simulink model "SOC_predict"  (R2023b)
settings: Solver=FixedStepDiscrete  StartTime=0.0  StopTime=timeVector(end)  FixedStep=stepSize  RelTol=1e-3
undefined symbols (not defined in the file): X_MAX, X_MIN
libraries: statsLibrary x1
settings Model: Creator=The MathWorks, Inc.  LastModifiedBy=The MathWorks, Inc.
settings OptimizationCC: BlockReduction=off  ConditionallyExecuteInputs=off  DefaultParameterBehavior=Inlined  InheritOutputTypeSmallerThanSingle=on
settings DebuggingCC: AlgebraicLoopMsg=error  InheritedTsInSrcMsg=none  SingleTaskRateTransMsg=error
settings HardwareCC: ProdBitPerPointer=32  ProdBitPerSizeT=32  ProdBitPerPtrDiffT=32  ProdLargestAtomicFloat=None  ProdIntDivRoundTo=Undefined  ProdEndianess=Unspecified  ProdWordSize=32  ProdHWDeviceType=ASIC/FPGA->ASIC/FPGA  TargetBitPerLong=64  TargetBitPerPointer=64  TargetBitPerSizeT=64  TargetBitPerPtrDiffT=64  TargetLongLongMode=on  TargetIntDivRoundTo=Zero  TargetEndianess=LittleEndian  TargetWordSize=64  TargetHWDeviceType=Custom Processor->MATLAB Host Computer  ProdEqTarget=off
settings ModelReferenceCC: EnableRefExpFcnMdlSchedulingChecks=on

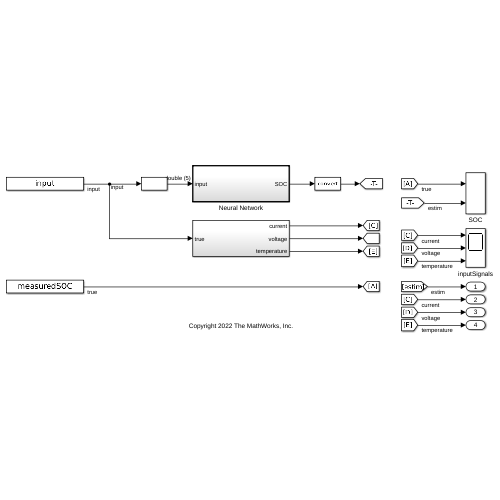
[thumbnail: Simulink's stored preview of the top-level diagram]
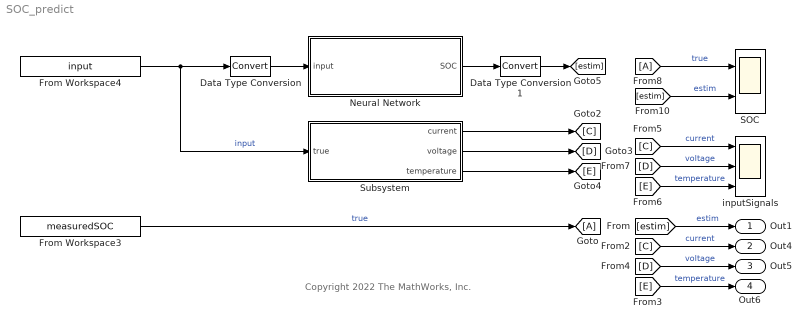
== system SOC_predict ==
  note: Copyright 2022 The MathWorks, Inc.
  Data Type Conversion : DataTypeConversion  SaturateOnIntegerOverflow=off  RndMeth=Floor
  Data Type Conversion1 : DataTypeConversion  SaturateOnIntegerOverflow=off  RndMeth=Floor
  From Workspace3 : FromWorkspace  VariableName=measuredSOC  SampleTime=-1
  From Workspace4 : FromWorkspace  VariableName=input  SampleTime=-1
  From8 : From
  Goto : Goto
  Neural Network : Subsystem  TreatAsAtomicUnit=on
  SOC : Scope  NumInputPorts=2
  Subsystem : Subsystem
  inputSignals : Scope  NumInputPorts=3
  Out1 : Outport
  Out4 : Outport  Port=2
  Out5 : Outport  Port=3
  Out6 : Outport  Port=4
  wires:
  Data Type Conversion1/1 -> [estim]
  Data Type Conversion/1 -> Neural Network/1(input)
  From Workspace4/1 -> Subsystem/1(true), Data Type Conversion/1  "input"
  [D] -> Out5/1  "voltage"
  [E] -> inputSignals/3  "temperature"
  [estim] -> SOC/2  "estim"
  From8/1 -> SOC/1  "true"
  [C] -> Out4/1  "current"
  [D] -> inputSignals/2  "voltage"
  [C] -> inputSignals/1  "current"
  From Workspace3/1 -> Goto/1  "true"
  Neural Network/1(SOC) -> Data Type Conversion1/1
  Subsystem/3(temperature) -> [E]
  [estim] -> Out1/1  "estim"
  Subsystem/1(current) -> [C]
  Subsystem/2(voltage) -> [D]
  [E] -> Out6/1  "temperature"

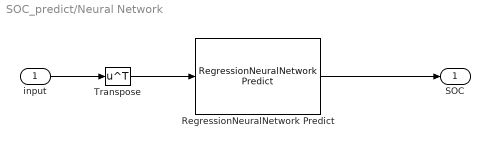
== system SOC_predict/Neural Network ==
  input : Inport  OutDataTypeStr=double  PortDimensions=[5]  SampleTime=10
  RegressionNeuralNetwork Predict : statsLibrary/Regression/RegressionNeuralNetwork Predict  TrainedLearner=nnetMdl  OutMin=[]  OutMax=[]  OutputLayerOutMin=[]  OutputLayerOutMax=[]  OutputLayerAdditionOutMin=[]  OutputLayerAdditionOutMax=[]  LayerSelector=Layer 1  Layer1OutMin=[]  Layer1OutMax=[]  Layer1AdditionOutMin=[]  Layer1AdditionOutMax=[]  Layer2OutMin=[]  Layer2OutMax=[]  Layer2AdditionOutMin=[]  Layer2AdditionOutMax=[]  Layer3OutMin=[]  Layer3OutMax=[]  Layer3AdditionOutMin=[]  Layer3AdditionOutMax=[]  Layer4OutMin=[]  Layer4OutMax=[]  Layer4AdditionOutMin=[]  Layer4AdditionOutMax=[]  Layer5OutMin=[]  Layer5OutMax=[]  Layer5AdditionOutMin=[]  Layer5AdditionOutMax=[]  Layer6OutMin=[]  Layer6OutMax=[]  Layer6AdditionOutMin=[]  Layer6AdditionOutMax=[]  Layer7OutMin=[]  Layer7OutMax=[]  Layer7AdditionOutMin=[]  Layer7AdditionOutMax=[]  Layer8OutMin=[]  Layer8OutMax=[]  Layer8AdditionOutMin=[]  Layer8AdditionOutMax=[]  Layer9OutMin=[]  Layer9OutMax=[]  Layer9AdditionOutMin=[]  Layer9AdditionOutMax=[]  Layer10OutMin=[]  Layer10OutMax=[]  Layer10AdditionOutMin=[]  Layer10AdditionOutMax=[]  Layer11OutMin=[]  Layer11OutMax=[]  Layer11AdditionOutMin=[]  Layer11AdditionOutMax=[]  StandardizedInputOutMin=[]  StandardizedInputOutMax=[]  NumHiddenLayers=1
  Transpose : Math  Operator=transpose
  SOC : Outport  SampleTime=10
  wires:
  input/1 -> Transpose/1
  RegressionNeuralNetwork Predict/1 -> SOC/1
  Transpose/1 -> RegressionNeuralNetwork Predict/1

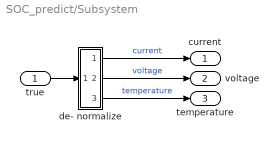
== system SOC_predict/Subsystem ==
  true : Inport
  de- normalize : Subsystem
  current : Outport
  voltage : Outport  Port=2
  temperature : Outport  Port=3
  wires:
  true/1 -> de- normalize/1(u)
  de- normalize/3(T) -> temperature/1  "temperature"
  de- normalize/1(I) -> current/1  "current"
  de- normalize/2(V) -> voltage/1  "voltage"

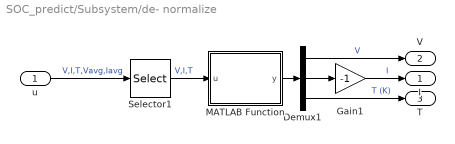
== system SOC_predict/Subsystem/de- normalize ==
  u : Inport
  Demux1 : Demux  Outputs=3
  Gain1 : Gain  Gain=-1
  MATLAB Function : MATLAB Function  TreatAsAtomicUnit=on
  Selector1 : Selector  InputPortWidth=5  IndexOptions=Index vector (dialog)  Indices=[1 2 3]  OutputSizes=1
  I : Outport
  V : Outport  Port=2
  T : Outport  Port=3
  wires:
  Gain1/1 -> I/1  "I"
  Selector1/1 -> MATLAB Function/1(u)  "V,I,T"
  Demux1/2 -> Gain1/1
  Demux1/1 -> V/1  "V"
  Demux1/3 -> T/1  "T (K)"
  MATLAB Function/1(y) -> Demux1/1
  u/1 -> Selector1/1  "V,I,T,Vavg,Iavg"

== matlab function SOC_predict/Subsystem/de- normalize/MATLAB Function ==
  data: u input; y output; X_MAX parameter; X_MIN parameter
function y = fcn(u, X_MAX, X_MIN)
y = (X_MAX-X_MIN).*u+X_MIN;
y(3) = y(3) + 273.15; % convert to K
